simulink library "FlatSatInterface_lib"  (R2018b)
settings: Solver=VariableStepAuto  StartTime=0.0  StopTime=10.0  RelTol=1e-3
undefined symbols (not defined in the file or in its folder): LF, mtq_dipole_body_Am2, rwa_torque_body_Nm, serial, simParams
libraries: instrumentlib x11, dspindex x2, dspsigattribs x1, actuator_control_bus x1
settings Model: Creator=aact_  LastModifiedBy=aact_

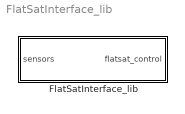
== system FlatSatInterface_lib ==
  FlatSatInterface_lib : Subsystem

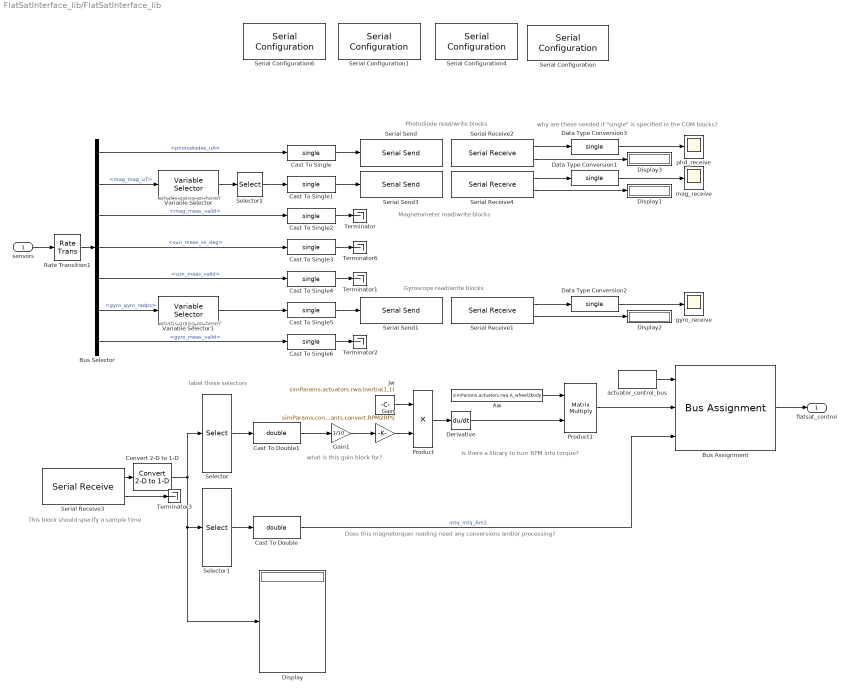
== system FlatSatInterface_lib/FlatSatInterface_lib ==
  note: what's going on here?
  note: Photodiode read/write blocks
  note: Does this magnetorquer reading need any conversions and/or processing?
  note: Is there a library to turn RPM into torque?
  note: label these selectors
  note: what is this gain block for?
  note: Magnetometer read/write blocks
  note: Gyroscope read/write blocks
  note: what's going on here?
  note: This block should specify a sample time
  note: why are these needed if "single" is specified in the COM blocks?
  sensors : Inport  OutDataTypeStr=Bus: sensor_bus
  Aw : Constant  Value=simParams.actuators.rwa.A_wheel2body  SampleTime=simParams.sample_time_s
  Bus Assignment : BusAssignment  AssignedSignals=rwa_torque_body_Nm,mtq_dipole_body_Am2
  Bus Selector : BusSelector  OutputSignals=photodiodes_uA,mag_mag_uT,mag_meas_valid,sun_meas_ss_deg,sun_meas_valid,gyro_gyro_radps,gyro_meas_valid
  Cast To Double : DataTypeConversion  OutDataTypeStr=double
  Cast To Double1 : DataTypeConversion  OutDataTypeStr=double
  Cast To Single{,1..6} (7 alike) : DataTypeConversion  OutDataTypeStr=single
  Convert 2-D to 1-D : dspsigattribs/Convert 2-D to 1-D
      settings: SourceProductName=DSP System Toolbox  SourceProductBaseCode=DS
  Data Type Conversion1 : DataTypeConversion  OutDataTypeStr=single
  Data Type Conversion2 : DataTypeConversion  OutDataTypeStr=single
  Data Type Conversion3 : DataTypeConversion  OutDataTypeStr=single
  Derivative : Derivative
  Display{,1..3} (4 alike) : Display
  Gain : Gain  Gain=simParams.constants.convert.RPM2RPS
  Gain1 : Gain  Gain=1/10
  Jw : Constant  Value=simParams.actuators.rwa.inertia(1,1)
  Product : Product
  Product1 : Product  Multiplication=Matrix(*)
  Rate Transition1 : RateTransition  OutPortSampleTime=fswParams.sample_time_s
  Selector : Selector  InputPortWidth=8  IndexOptions=Index vector (dialog)  Indices=[4 5 6 7]  OutputSizes=1
  Selector1 : Selector  InputPortWidth=8  IndexOptions=Index vector (dialog)  Indices=[1 2 3]  OutputSizes=1
  Selector2 : Selector  InputPortWidth=3  IndexOptions=Index vector (dialog)  Indices=[1 3 2]  OutputSizes=1
  Serial Configuration : instrumentlib/Serial Configuration  Priority=-200000  ComPortMenu=<Please select a port...>  ComPort=COM3  ObjConstructor=serial('COM3');  BaudRate=115200  DataBits=8  Parity=none  StopBits=1  FlowControl=none  Timeout=10  ByteOrder=LittleEndian
  Serial Configuration1 : instrumentlib/Serial Configuration  Priority=-200000  ComPortMenu=COM9  ComPort=COM9  ObjConstructor=serial('COM9');  BaudRate=115200  DataBits=8  Parity=none  StopBits=1  FlowControl=none  Timeout=10  ByteOrder=BigEndian
  Serial Configuration4 : instrumentlib/Serial Configuration  Priority=-200000  ComPortMenu=COM10  ComPort=COM10  ObjConstructor=serial('COM10');  BaudRate=115200  DataBits=8  Parity=none  StopBits=1  FlowControl=none  Timeout=10  ByteOrder=BigEndian
  Serial Configuration6 : instrumentlib/Serial Configuration  Priority=-200000  ComPortMenu=COM11  ComPort=COM11  ObjConstructor=serial('COM11');  BaudRate=115200  DataBits=8  Parity=none  StopBits=1  FlowControl=none  Timeout=10  ByteOrder=BigEndian
  Serial Receive1 : instrumentlib/Serial Receive  ComPortMenu=COM10  ComPort=COM10  ObjConstructor=serial('COM10');  Terminator=<none>  DataSize="[3  1]"  DataType=single  EnableBlockingMode=off  ActionDataUnavailable=Output last received value  CustomValue=0  SampleTime=0.25
  Serial Receive2 : instrumentlib/Serial Receive  ComPortMenu=COM11  ComPort=COM11  ObjConstructor=serial('COM11');  Terminator=LF ('\n')  DataSize="[5  1]"  DataType=single  EnableBlockingMode=off  ActionDataUnavailable=Output last received value  CustomValue=0  SampleTime=0.25
  Serial Receive3 : instrumentlib/Serial Receive  ComPortMenu=<Please select a port...>  ComPort=COM3  ObjConstructor=serial('COM3');  Terminator=<none>  DataSize="[8  1]"  DataType=single  EnableBlockingMode=off  ActionDataUnavailable=Output last received value  CustomValue=0  SampleTime=-1
  Serial Receive4 : instrumentlib/Serial Receive  ComPortMenu=COM9  ComPort=COM9  ObjConstructor=serial('COM9');  Terminator=<none>  DataSize="[3  1]"  DataType=single  EnableBlockingMode=off  ActionDataUnavailable=Output last received value  CustomValue=0  SampleTime=0.25
  Serial Send : instrumentlib/Serial Send  ComPortMenu=COM11  ComPort=COM11  ObjConstructor=serial('COM11');  Terminator=LF ('\n')  EnableBlockingMode=off
  Serial Send1 : instrumentlib/Serial Send  ComPortMenu=COM10  ComPort=COM10  ObjConstructor=serial('COM10');  Terminator=<none>  EnableBlockingMode=off
  Serial Send3 : instrumentlib/Serial Send  ComPortMenu=COM9  ComPort=COM9  ObjConstructor=serial('COM9');  Terminator=<none>  EnableBlockingMode=off
  Terminator{,1..3,6} (5 alike) : Terminator
  Variable Selector : dspindex/Variable Selector  NumInputs=1  rowsOrCols=Columns  IdxMode=Fixed  Elements=[3]  ZerOneIdxMode=One-based  errmode=Clip Index  FillMode=on  FillValues=0
  Variable Selector1 : dspindex/Variable Selector  NumInputs=1  rowsOrCols=Columns  IdxMode=Fixed  Elements=[1]  ZerOneIdxMode=One-based  errmode=Clip Index  FillMode=on  FillValues=0
  actuator_control_bus : actuator_control_bus/actuator_control_bus  SystemSampleTime=-1
  gyro_receive : Scope
  mag_receive : Scope
  phd_receive : Scope
  flatsat_control : Outport  OutDataTypeStr=Bus: actuator_control
  wires:
  Bus Selector/7 -> Cast To Single6/1  "<gyro_meas_valid>"
  Cast To Double/1 -> Bus Assignment/3  "mtq_mtq_Am2"
  Cast To Single4/1 -> Terminator1/1
  Derivative/1 -> Product1/2
  Serial Receive3/1 -> Convert 2-D to 1-D/1
  Bus Selector/5 -> Cast To Single4/1  "<sun_meas_valid>"
  Bus Selector/4 -> Cast To Single3/1  "<sun_meas_ss_deg>"
  Aw/1 -> Product1/1
  Product1/1 -> Bus Assignment/2
  Selector1/1 -> Cast To Double/1
  Bus Selector/1 -> Cast To Single/1  "<photodiodes_uA>"
  Jw/1 -> Product/1
  Rate Transition1/1 -> Bus Selector/1
  Serial Receive4/1 -> Data Type Conversion1/1
  Serial Receive2/2 -> Display3/1
  Bus Selector/6 -> Variable Selector1/1  "<gyro_gyro_radps>"
  Product/1 -> Derivative/1
  Cast To Single1/1 -> Serial Send3/1
  actuator_control_bus/1 -> Bus Assignment/1
  sensors/1 -> Rate Transition1/1
  Convert 2-D to 1-D/1 -> Display/1, Selector1/1, Selector/1
  Data Type Conversion3/1 -> phd_receive/1
  Cast To Single/1 -> Serial Send/1
  Data Type Conversion1/1 -> mag_receive/1
  Gain1/1 -> Gain/1
  Selector2/1 -> Cast To Single1/1
  Bus Selector/3 -> Cast To Single2/1  "<mag_meas_valid>"
  Variable Selector/1 -> Selector2/1
  Bus Selector/2 -> Variable Selector/1  "<mag_mag_uT>"
  Cast To Single5/1 -> Serial Send1/1
  Selector/1 -> Cast To Double1/1
  Bus Assignment/1 -> flatsat_control/1
  Serial Receive1/1 -> Data Type Conversion2/1
  Serial Receive3/2 -> Terminator3/1
  Serial Receive2/1 -> Data Type Conversion3/1
  Variable Selector1/1 -> Cast To Single5/1
  Cast To Single3/1 -> Terminator6/1
  Data Type Conversion2/1 -> gyro_receive/1
  Gain/1 -> Product/2
  Cast To Single6/1 -> Terminator2/1
  Serial Receive1/2 -> Display2/1
  Cast To Single2/1 -> Terminator/1
  Serial Receive4/2 -> Display1/1
  Cast To Double1/1 -> Gain1/1
